simulink model "zn"  (R2021a)
settings: Solver=VariableStepAuto  StartTime=0.0  StopTime=8500  RelTol=1e-3
undefined symbols (not defined in the file or in its folder): se
settings Model: Creator=dell  LastModifiedBy=dell

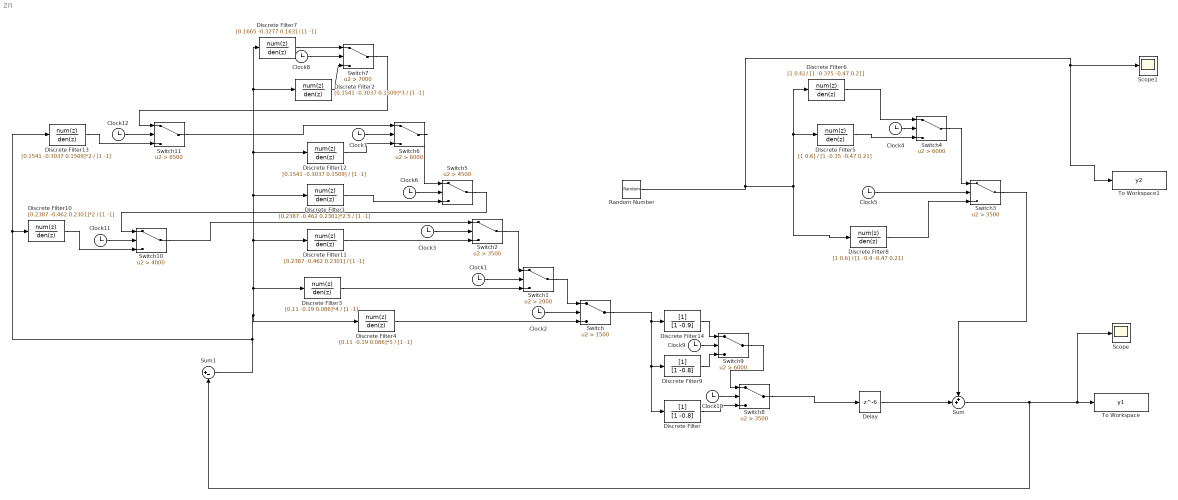
== system zn ==
  Clock{1..12} (12 alike) : Clock
  Delay : Delay  DelayLength=6  SampleTime=0.1
  Discrete Filter : DiscreteFilter  Denominator=[1 -0.8]  SampleTime=0.1
  Discrete Filter1 : DiscreteFilter  Numerator=[0.2387 -0.462 0.2301]*2.5  Denominator=[1 -1]  SampleTime=0.1
  Discrete Filter10 : DiscreteFilter  Numerator=[0.2387 -0.462 0.2301]*2  Denominator=[1 -1]  SampleTime=0.1
  Discrete Filter11 : DiscreteFilter  Numerator=[0.2387 -0.462 0.2301]  Denominator=[1 -1]  SampleTime=0.1
  Discrete Filter12 : DiscreteFilter  Numerator=[0.1541 -0.3037 0.1509]  Denominator=[1 -1]  SampleTime=0.1
  Discrete Filter13 : DiscreteFilter  Numerator=[0.1541 -0.3037 0.1509]*2  Denominator=[1 -1]  SampleTime=0.1
  Discrete Filter14 : DiscreteFilter  Denominator=[1 -0.9]  SampleTime=0.1
  Discrete Filter2 : DiscreteFilter  Numerator=[0.1541 -0.3037 0.1509]*3  Denominator=[1 -1]  SampleTime=0.1
  Discrete Filter3 : DiscreteFilter  Numerator=[0.11 -0.19 0.086]*4  Denominator=[1 -1]  SampleTime=0.1
  Discrete Filter4 : DiscreteFilter  Numerator=[0.11 -0.19 0.086]*5  Denominator=[1 -1]  SampleTime=0.1
  Discrete Filter5 : DiscreteFilter  Numerator=[1 0.6]  Denominator=[1 -0.35 -0.47 0.21]  SampleTime=0.1
  Discrete Filter6 : DiscreteFilter  Numerator=[1 0.6]  Denominator=[1 -0.375 -0.47 0.21]  SampleTime=0.1
  Discrete Filter7 : DiscreteFilter  Numerator=[0.1665 -0.3277 0.163]  Denominator=[1 -1]  SampleTime=0.1
  Discrete Filter8 : DiscreteFilter  Numerator=[1 0.6]  Denominator=[1 -0.4 -0.47 0.21]  SampleTime=0.1
  Discrete Filter9 : DiscreteFilter  Denominator=[1 -0.8]  SampleTime=0.1
  Random Number : RandomNumber  Seed=se  SampleTime=0.1
  Scope : Scope
  Scope1 : Scope
  Sum : Sum  Inputs=++|
  Sum1 : Sum  Inputs=|+-
  Switch : Switch  Criteria=u2 > Threshold  Threshold=1500
  Switch1 : Switch  Criteria=u2 > Threshold  Threshold=2000
  Switch10 : Switch  Criteria=u2 > Threshold  Threshold=4000
  Switch11 : Switch  Criteria=u2 > Threshold  Threshold=6500
  Switch2 : Switch  Criteria=u2 > Threshold  Threshold=3500
  Switch3 : Switch  Criteria=u2 > Threshold  Threshold=3500
  Switch4 : Switch  Criteria=u2 > Threshold  Threshold=6000
  Switch5 : Switch  Criteria=u2 > Threshold  Threshold=4500
  Switch6 : Switch  Criteria=u2 > Threshold  Threshold=6000
  Switch7 : Switch  Criteria=u2 > Threshold  Threshold=7000
  Switch8 : Switch  Criteria=u2 > Threshold  Threshold=3500
  Switch9 : Switch  Criteria=u2 > Threshold  Threshold=6000
  To Workspace : ToWorkspace  VariableName=y1  SampleTime=0.1
  To Workspace1 : ToWorkspace  VariableName=y2  SampleTime=0.1
  wires:
  Clock6/1 -> Switch5/2
  Clock1/1 -> Switch1/2
  Discrete Filter8/1 -> Switch3/3
  Discrete Filter5/1 -> Switch4/3
  Discrete Filter4/1 -> Switch/3
  Random Number/1 -> To Workspace1/1, Scope1/1, Discrete Filter8/1, Discrete Filter5/1, Discrete Filter6/1
  Sum/1 -> Scope/1, To Workspace/1, Sum1/2
  Switch6/1 -> Switch5/1
  Discrete Filter3/1 -> Switch1/3
  Clock4/1 -> Switch4/2
  Delay/1 -> Sum/2
  Sum1/1 -> Discrete Filter13/1, Discrete Filter10/1, Discrete Filter2/1, Discrete Filter7/1, Discrete Filter12/1, Discrete Filter1/1, Discrete Filter11/1, Discrete Filter3/1, Discrete Filter4/1
  Switch4/1 -> Switch3/1
  Clock7/1 -> Switch6/2
  Clock3/1 -> Switch2/2
  Discrete Filter11/1 -> Switch2/3
  Clock2/1 -> Switch/2
  Discrete Filter6/1 -> Switch4/1
  Switch2/1 -> Switch1/1
  Switch3/1 -> Sum/1
  Discrete Filter12/1 -> Switch6/3
  Switch1/1 -> Switch/1
  Clock5/1 -> Switch3/2
  Clock8/1 -> Switch7/2
  Discrete Filter7/1 -> Switch7/1
  Discrete Filter2/1 -> Switch7/3
  Discrete Filter1/1 -> Switch5/3
  Discrete Filter/1 -> Switch8/3
  Clock9/1 -> Switch9/2
  Clock10/1 -> Switch8/2
  Switch9/1 -> Switch8/1
  Discrete Filter14/1 -> Switch9/1
  Switch/1 -> Discrete Filter14/1, Discrete Filter9/1, Discrete Filter/1
  Discrete Filter9/1 -> Switch9/3
  Switch8/1 -> Delay/1
  Clock11/1 -> Switch10/2
  Clock12/1 -> Switch11/2
  Discrete Filter10/1 -> Switch10/3
  Switch10/1 -> Switch2/1
  Switch5/1 -> Switch10/1
  Discrete Filter13/1 -> Switch11/3
  Switch11/1 -> Switch6/1
  Switch7/1 -> Switch11/1
